simulink model "casperdemo"  (Simulink 6.2)
settings: Solver=ode45  StartTime=0.0  StopTime=16384  RelTol=1e-3
libraries: xbsIndex_r3 x1645, casper_library x163, testbench_lib x15, xps_library x1
(part 7 of 12)

== system casperdemo/Real FFT and Real PFB/fft_biplex_real_4x/biplex_core/fft_stage_3 ==
  in1 : Inport  Port=1  LatchInput=off
  in2 : Inport  Port=2  LatchInput=off
  of_in : Inport  Port=3  LatchInput=off
  sync : Inport  Port=4  LatchInput=off
  shift : Inport  Port=5  LatchInput=off
  Counter : xbsIndex_r3/Counter  cnt_type=Free Running  n_bits=FFTSize-FFTStage+1  bin_pt=0  arith_type=Unsigned  start_count=0  cnt_to=Inf  cnt_by_val=1  operation=Up  explicit_period=off  period=1  load_pin=off  rst=on  en=off  dbl_ovrd=off  show_param=off  use_rpm=off  gen_core=on
      settings: xl_area=[0, 0, 0, 0, 0, 0, 0]
  Delay : xbsIndex_r3/Delay  latency=1  reg_retiming=off  explicit_period=off  period=1  en=off  accept_only_valid=off  init_zero=on  dbl_ovrd=off  show_param=off
      settings: xl_area=[0, 0, 0, 0, 0, 0, 0]
  Logical1 : xbsIndex_r3/Logical  logical_function=OR  inputs=2  precision=Full  arith_type=Unsigned  n_bits=8  bin_pt=2  align_bp=on  latency=1  explicit_period=on  period=1  en=off  dbl_ovrd=off  show_param=off
      settings: xl_area=[0, 0, 0, 0, 0, 0, 0]
  Mux : xbsIndex_r3/Mux  inputs=2  precision=Full  arith_type="Signed  (2's comp)"  n_bits=8  bin_pt=2  quantization=Truncate  overflow=Wrap  latency=1  explicit_period=off  period=1  en=off  dbl_ovrd=off  show_param=off  mux_type=off  use_rpm=off  gen_core=on
      settings: xl_area=[0, 0, 0, 0, 0, 0, 0]
  Mux1 : xbsIndex_r3/Mux  inputs=2  precision=Full  arith_type="Signed  (2's comp)"  n_bits=8  bin_pt=2  quantization=Truncate  overflow=Wrap  latency=1  explicit_period=off  period=1  en=off  dbl_ovrd=off  show_param=off  mux_type=off  use_rpm=off  gen_core=on
      settings: xl_area=[0, 0, 0, 0, 0, 0, 0]
  Slice : xbsIndex_r3/Slice  Orientation=up  mode=Lower Bit Location + Width  nbits=1  bit1=-(FFTStage - 1)  base1=MSB of Input  bit0=FFTStage - 1  base0=LSB of Input  boolean_output=on  explicit_period=off  period=1  dbl_ovrd=off
  Slice1 : xbsIndex_r3/Slice  mode=Upper Bit Location + Width  nbits=1  bit1=0  base1=MSB of Input  bit0=0  base0=LSB of Input  boolean_output=off  explicit_period=off  period=1  dbl_ovrd=off
  butterfly_direct : Subsystem  AncestorBlock=casper_library/FFTs/butterfly_direct  mask(butterfly_direct){FFTSize=4, Coeffs=[0 1 2 3], StepPeriod=1, BitWidth=18, add_latency=2, mult_latency=3, bram_latency=2, use_bram=0, quantization=Truncate, overflow=Wrap}
      mask prompts: FFTSize "Size of FFT: (2^?)"; Coeffs "Coefficients: (0 to 2^(FFTSize-1)-1)"; StepPeriod "Coefficient Step Period: (2^?)"; BitWidth "Output Bitwidth:"; add_latency "Add Latency"; mult_latency "Mult Latency"; bram_latency "BRAM Latency"; use_bram "Store Coefficients in BRAM"; quantization "Quantization Behavior"; overflow "Overflow Behavior"
      mask init: same as casperdemo/Complex FFT and PFB with multiple simultaneous inputs/fft/fft_direct/butterfly1_0
      settings: AttributesFormatString=|
      | FFTSize=4, Coeffs=[0  1  2  3],
      |  StepPeriod=1, BitWidth=18
      mask StyleString: edit,edit,edit,edit,edit,edit,edit,edit,popup(Truncate|Round  (unbiased: +/- Inf)|Round  (unbiased: Even Values)),popup(Wrap|Saturate|Error)
  delay_b : Subsystem  BlockChoice=delay_slr
      link override delay_bram: bram_latency=bram_latency  DelayLen=2^(FFTSize-FFTStage)
      link override delay_slr: DelayLen=2^(FFTSize-FFTStage)
      settings: AttributesFormatString=%<BlockChoice>  TemplateBlock=casper_library/Delays/delay  MemberBlocks=delay_bram,delay_slr
  delay_f : Subsystem  BlockChoice=delay_slr
      link override delay_bram: bram_latency=bram_latency  DelayLen=2^(FFTSize-FFTStage)
      link override delay_slr: DelayLen=2^(FFTSize-FFTStage)
      settings: AttributesFormatString=%<BlockChoice>  TemplateBlock=casper_library/Delays/delay  MemberBlocks=delay_bram,delay_slr
  sync_delay : casper_library/Delays/sync_delay  DelayLen=2^(FFTSize - FFTStage)
      link override Constant: equ=P=C
      link override Constant1: equ=P=C
      link override Constant2: equ=P=C
      link override Constant3: equ=P=C
  out1 : Outport
  out2 : Outport  Port=2
  of : Outport  Port=3
  sync_out : Outport  Port=4
  wires:
  butterfly_direct/4(sync_out) -> sync_out/1
  butterfly_direct/1(a+bw) -> out1/1
  butterfly_direct/2(a-bw) -> out2/1
  butterfly_direct/3(of) -> Logical1/1
  Slice/1 -> butterfly_direct/4(shift)
  sync_delay/1 -> butterfly_direct/3(sync)
  delay_b/1(Out1) -> butterfly_direct/1(a)
  in2/1 -> delay_f/1(In1)
  Slice1/1 -> Mux1/1, Mux/1
  in1/1 -> Mux1/2, Mux/3
  delay_f/1(Out1) -> Mux/2, Mux1/3
  Mux1/1 -> delay_b/1(In1)
  Mux/1 -> butterfly_direct/2(b)
  Counter/1 -> Slice1/1
  sync/1 -> Delay/1, Counter/1
  Delay/1 -> sync_delay/1
  Logical1/1 -> of/1
  of_in/1 -> Logical1/2
  shift/1 -> Slice/1

== system casperdemo/Real FFT and Real PFB/fft_biplex_real_4x/biplex_core/fft_stage_4 ==
  in1 : Inport  Port=1  LatchInput=off
  in2 : Inport  Port=2  LatchInput=off
  of_in : Inport  Port=3  LatchInput=off
  sync : Inport  Port=4  LatchInput=off
  shift : Inport  Port=5  LatchInput=off
  Counter : xbsIndex_r3/Counter  cnt_type=Free Running  n_bits=FFTSize-FFTStage+1  bin_pt=0  arith_type=Unsigned  start_count=0  cnt_to=Inf  cnt_by_val=1  operation=Up  explicit_period=off  period=1  load_pin=off  rst=on  en=off  dbl_ovrd=off  show_param=off  use_rpm=off  gen_core=on
      settings: xl_area=[0, 0, 0, 0, 0, 0, 0]
  Delay : xbsIndex_r3/Delay  latency=1  reg_retiming=off  explicit_period=off  period=1  en=off  accept_only_valid=off  init_zero=on  dbl_ovrd=off  show_param=off
      settings: xl_area=[0, 0, 0, 0, 0, 0, 0]
  Logical1 : xbsIndex_r3/Logical  logical_function=OR  inputs=2  precision=Full  arith_type=Unsigned  n_bits=8  bin_pt=2  align_bp=on  latency=1  explicit_period=on  period=1  en=off  dbl_ovrd=off  show_param=off
      settings: xl_area=[0, 0, 0, 0, 0, 0, 0]
  Mux : xbsIndex_r3/Mux  inputs=2  precision=Full  arith_type="Signed  (2's comp)"  n_bits=8  bin_pt=2  quantization=Truncate  overflow=Wrap  latency=1  explicit_period=off  period=1  en=off  dbl_ovrd=off  show_param=off  mux_type=off  use_rpm=off  gen_core=on
      settings: xl_area=[0, 0, 0, 0, 0, 0, 0]
  Mux1 : xbsIndex_r3/Mux  inputs=2  precision=Full  arith_type="Signed  (2's comp)"  n_bits=8  bin_pt=2  quantization=Truncate  overflow=Wrap  latency=1  explicit_period=off  period=1  en=off  dbl_ovrd=off  show_param=off  mux_type=off  use_rpm=off  gen_core=on
      settings: xl_area=[0, 0, 0, 0, 0, 0, 0]
  Slice : xbsIndex_r3/Slice  Orientation=up  mode=Lower Bit Location + Width  nbits=1  bit1=-(FFTStage - 1)  base1=MSB of Input  bit0=FFTStage - 1  base0=LSB of Input  boolean_output=on  explicit_period=off  period=1  dbl_ovrd=off
  Slice1 : xbsIndex_r3/Slice  mode=Upper Bit Location + Width  nbits=1  bit1=0  base1=MSB of Input  bit0=0  base0=LSB of Input  boolean_output=off  explicit_period=off  period=1  dbl_ovrd=off
  butterfly_direct : Subsystem  AncestorBlock=casper_library/FFTs/butterfly_direct  mask(butterfly_direct){FFTSize=4, Coeffs=[0 1 2 3 4 5 6 7], StepPeriod=0, BitWidth=18, add_latency=2, mult_latency=3, bram_latency=2, use_bram=0, quantization=Truncate, overflow=Wrap}
      mask prompts: FFTSize "Size of FFT: (2^?)"; Coeffs "Coefficients: (0 to 2^(FFTSize-1)-1)"; StepPeriod "Coefficient Step Period: (2^?)"; BitWidth "Output Bitwidth:"; add_latency "Add Latency"; mult_latency "Mult Latency"; bram_latency "BRAM Latency"; use_bram "Store Coefficients in BRAM"; quantization "Quantization Behavior"; overflow "Overflow Behavior"
      mask init: same as casperdemo/Complex FFT and PFB with multiple simultaneous inputs/fft/fft_direct/butterfly1_0
      settings: AttributesFormatString=|
      | FFTSize=4, Coeffs=[0  1  2  3  4  5  6  7],
      |  StepPeriod=0, BitWidth=18
      mask StyleString: edit,edit,edit,edit,edit,edit,edit,edit,popup(Truncate|Round  (unbiased: +/- Inf)|Round  (unbiased: Even Values)),popup(Wrap|Saturate|Error)
  delay_b : Subsystem  BlockChoice=delay_slr
      link override delay_bram: bram_latency=bram_latency  DelayLen=2^(FFTSize-FFTStage)
      link override delay_slr: DelayLen=2^(FFTSize-FFTStage)
      settings: AttributesFormatString=%<BlockChoice>  TemplateBlock=casper_library/Delays/delay  MemberBlocks=delay_bram,delay_slr
  delay_f : Subsystem  BlockChoice=delay_slr
      link override delay_bram: bram_latency=bram_latency  DelayLen=2^(FFTSize-FFTStage)
      link override delay_slr: DelayLen=2^(FFTSize-FFTStage)
      settings: AttributesFormatString=%<BlockChoice>  TemplateBlock=casper_library/Delays/delay  MemberBlocks=delay_bram,delay_slr
  sync_delay : casper_library/Delays/sync_delay  DelayLen=2^(FFTSize - FFTStage)
      link override Constant: equ=P=C
      link override Constant1: equ=P=C
      link override Constant2: equ=P=C
      link override Constant3: equ=P=C
  out1 : Outport
  out2 : Outport  Port=2
  of : Outport  Port=3
  sync_out : Outport  Port=4
  wires:
  butterfly_direct/4(sync_out) -> sync_out/1
  butterfly_direct/1(a+bw) -> out1/1
  butterfly_direct/2(a-bw) -> out2/1
  butterfly_direct/3(of) -> Logical1/1
  Slice/1 -> butterfly_direct/4(shift)
  sync_delay/1 -> butterfly_direct/3(sync)
  delay_b/1(Out1) -> butterfly_direct/1(a)
  in2/1 -> delay_f/1(In1)
  Slice1/1 -> Mux1/1, Mux/1
  in1/1 -> Mux1/2, Mux/3
  delay_f/1(Out1) -> Mux/2, Mux1/3
  Mux1/1 -> delay_b/1(In1)
  Mux/1 -> butterfly_direct/2(b)
  Counter/1 -> Slice1/1
  sync/1 -> Delay/1, Counter/1
  Delay/1 -> sync_delay/1
  Logical1/1 -> of/1
  of_in/1 -> Logical1/2
  shift/1 -> Slice/1

== system casperdemo/Real FFT and Real PFB/pfb_fir_real/pol1_in1_first_tap/delay ==
  In1 : Inport  Port=1  LatchInput=off
  delay_bram : casper_library/Delays/delay_bram  DelayLen=2^(PFBSize-n_inputs)  bram_latency=bram_latency
  Out1 : Outport
  wires:
  In1/1 -> delay_bram/1
  delay_bram/1 -> Out1/1

== system casperdemo/Real FFT and Real PFB/pfb_fir_real/pol1_in1_first_tap/pfb_coeff_gen ==
  din : Inport  Port=1  LatchInput=off
  sync : Inport  Port=2  LatchInput=off
  Concat : xbsIndex_r3/Concat  num_inputs=4  explicit_period=off  period=1  dbl_ovrd=off
  Counter : xbsIndex_r3/Counter  cnt_type=Free Running  n_bits=4  bin_pt=0  arith_type=Unsigned  start_count=0  cnt_to=Inf  cnt_by_val=1  operation=Up  explicit_period=on  period=1  load_pin=off  rst=on  en=off  dbl_ovrd=off  show_param=off  use_rpm=on  gen_core=off
      settings: xl_area=[0, 0, 0, 0, 0, 0, 0]
  Delay : xbsIndex_r3/Delay  latency=bram_latency+1  reg_retiming=off  explicit_period=off  period=1  en=off  accept_only_valid=off  init_zero=on  dbl_ovrd=off  show_param=off
      settings: xl_area=[0, 0, 0, 0, 0, 0, 0]
  Delay1 : xbsIndex_r3/Delay  latency=3  reg_retiming=off  explicit_period=off  period=1  en=off  accept_only_valid=off  init_zero=on  dbl_ovrd=off  show_param=off
      settings: xl_area=[0, 0, 0, 0, 0, 0, 0]
  ROM1 : xbsIndex_r3/ROM  depth=16  initVector=[-3.1185374660155e-018 -0.00263735909580334 -0.00578984434733957 -0.0097994723321974 -0.0149350827451364 -0.021332873381912 -0.0289429297169117 -0.0374871259095755 -0.0464331498505763 -0.054988365242619 -0.0621158358774173 -0.0665731978343029 -0.0669732935066947 -0.0618637102387744 -0.0498207328553067 -0.0295518537627434]  arith_type="Signed  (2's comp)"  n_bits=8  bin_pt=7  latency=2  init_zero=on  explicit_period=off  period=1  rst=off  init_reg=0  en=off  dbl_ovrd=off  show_param=on  distributed_mem=on  use_rpm=on  gen_core=off
      settings: xl_area=[0, 0, 0, 0, 0, 0, 0]
  ROM2 : xbsIndex_r3/ROM  depth=16  initVector=[2.14971748489781e-017 0.039557878919974 0.0894252110701411 0.149419992109658 0.218834505309546 0.29642479737618 0.380432267164858 0.468637627642037 0.558445322336343 0.646994370487006 0.731289732081715 0.808346763068111 0.875340286111191 0.929749314368444 0.969488576724053 0.993018702047571]  arith_type="Signed  (2's comp)"  n_bits=8  bin_pt=7  latency=2  init_zero=on  explicit_period=off  period=1  rst=off  init_reg=0  en=off  dbl_ovrd=off  show_param=on  distributed_mem=on  use_rpm=on  gen_core=off
      settings: xl_area=[0, 0, 0, 0, 0, 0, 0]
  ROM3 : xbsIndex_r3/ROM  depth=16  initVector=[0.999428183760704 0.988481980811812 0.960633699526478 0.917000599560915 0.859303017901024 0.789772045316812 0.711031265694996 0.625959945208598 0.537546129240986 0.448738600765768 0.36230654625236 0.280715079012005 0.20602354182225 0.139811844485469 0.0831381115043222 0.0365287647378851]  arith_type="Signed  (2's comp)"  n_bits=8  bin_pt=7  latency=2  init_zero=on  explicit_period=off  period=1  rst=off  init_reg=0  en=off  dbl_ovrd=off  show_param=off  distributed_mem=on  use_rpm=on  gen_core=off
      settings: xl_area=[0, 0, 0, 0, 0, 0, 0]
  ROM4 : xbsIndex_r3/ROM  depth=16  initVector=[1.9710098464648e-017 -0.0268924122607391 -0.0449798239071789 -0.0553900832155681 -0.0594466434903448 -0.0585648122922967 -0.0541523577793221 -0.0475209911960375 -0.0398141063792136 -0.0319546763151778 -0.0246155042127458 -0.0182122364356803 -0.0129178040136007 -0.00869539776353592 -0.00534581149262307 -0.00256409509972699]  arith_type="Signed  (2's comp)"  n_bits=8  bin_pt=7  latency=2  init_zero=on  explicit_period=off  period=1  rst=off  init_reg=0  en=off  dbl_ovrd=off  show_param=off  distributed_mem=on  use_rpm=on  gen_core=off
      settings: xl_area=[0, 0, 0, 0, 0, 0, 0]
  Register : xbsIndex_r3/Register  init=0  reg_only_valid=off  explicit_period=off  period=1  rst=off  en=off  out_en=off  dbl_ovrd=off  show_param=off
      settings: xl_area=[0, 0, 0, 0, 0, 0, 0]
  Reinterpret{1..4} (4 alike) : xbsIndex_r3/Reinterpret  force_arith_type=on  arith_type=Unsigned  force_bin_pt=on  bin_pt=0  force_valid=on
  dout : Outport
  sync_out : Outport  Port=2
  coeff : Outport  Port=3
  wires:
  din/1 -> Delay1/1
  Delay1/1 -> dout/1
  sync/1 -> Counter/1, Delay/1
  Delay/1 -> sync_out/1
  Concat/1 -> Register/1
  Register/1 -> coeff/1
  Counter/1 -> ROM1/1, ROM2/1, ROM3/1, ROM4/1
  ROM1/1 -> Reinterpret1/1
  Reinterpret1/1 -> Concat/1
  ROM2/1 -> Reinterpret2/1
  Reinterpret2/1 -> Concat/2
  ROM3/1 -> Reinterpret3/1
  Reinterpret3/1 -> Concat/3
  ROM4/1 -> Reinterpret4/1
  Reinterpret4/1 -> Concat/4

== system casperdemo/Real FFT and Real PFB/pfb_fir_real/pol1_in1_last_tap/pfb_real_add_tree ==
  din : Inport  Port=1  LatchInput=off
  sync : Inport  Port=2  LatchInput=off
  Reint{0..3} (4 alike) : xbsIndex_r3/Reinterpret  force_arith_type=on  arith_type="Signed  (2's comp)"  force_bin_pt=on  bin_pt=CoeffBitWidth + BitWidthIn - 2  force_valid=on
  Slice0 : xbsIndex_r3/Slice  mode=Upper Bit Location + Width  nbits=CoeffBitWidth + BitWidthIn  bit1=-0*(CoeffBitWidth + BitWidthIn)  base1=MSB of Input  bit0=0  base0=MSB of Input  boolean_output=off  explicit_period=off  period=1  dbl_ovrd=off
  Slice1 : xbsIndex_r3/Slice  mode=Upper Bit Location + Width  nbits=CoeffBitWidth + BitWidthIn  bit1=-1*(CoeffBitWidth + BitWidthIn)  base1=MSB of Input  bit0=0  base0=MSB of Input  boolean_output=off  explicit_period=off  period=1  dbl_ovrd=off
  Slice2 : xbsIndex_r3/Slice  mode=Upper Bit Location + Width  nbits=CoeffBitWidth + BitWidthIn  bit1=-2*(CoeffBitWidth + BitWidthIn)  base1=MSB of Input  bit0=0  base0=MSB of Input  boolean_output=off  explicit_period=off  period=1  dbl_ovrd=off
  Slice3 : xbsIndex_r3/Slice  mode=Upper Bit Location + Width  nbits=CoeffBitWidth + BitWidthIn  bit1=-3*(CoeffBitWidth + BitWidthIn)  base1=MSB of Input  bit0=0  base0=MSB of Input  boolean_output=off  explicit_period=off  period=1  dbl_ovrd=off
  adder_tree1 : Subsystem  AncestorBlock=casper_library/Misc/adder_tree  mask(adder_tree){n_inputs=4, latency=1}
      mask prompts: n_inputs "Number of Inputs"; latency "Add Latency"
      mask help: Sums all inputs using a tree of adds and delays.
      mask init:
      | adder_tree_init(gcb, ...
      |     'n_inputs', n_inputs, ...
      |     'latency', latency);
      settings: AttributesFormatString=latency 2
      mask Help: eval('xlWeb([getenv(''MLIB_ROOT''), ''\doc\html\sp_adder_tree\sp_adder_tree.html''])')
  convert1 : xbsIndex_r3/Convert  arith_type="Signed  (2's comp)"  n_bits=BitWidthOut  bin_pt=BitWidthOut-1  quantization=Truncate  overflow=Saturate  latency=add_latency  explicit_period=off  period=1  dbl_ovrd=off  show_param=off  inserted_by_tool=off  pipeline=off
      settings: xl_area=[0, 0, 0, 0, 0, 0, 0]
  delay1 : xbsIndex_r3/Delay  latency=1  reg_retiming=off  explicit_period=off  period=1  en=off  accept_only_valid=off  init_zero=on  dbl_ovrd=off  show_param=off
      settings: xl_area=[0, 0, 0, 0, 0, 0, 0]
  scale1 : xbsIndex_r3/Scale  scale_factor=-3  explicit_period=off  period=1  dbl_ovrd=off
  dout : Outport
  sync_out : Outport  Port=2
  wires:
  adder_tree1/2(dout) -> scale1/1
  scale1/1 -> convert1/1
  convert1/1 -> dout/1
  sync/1 -> adder_tree1/1(sync)
  adder_tree1/1(sync_out) -> delay1/1
  delay1/1 -> sync_out/1
  din/1 -> Slice0/1, Slice1/1, Slice2/1, Slice3/1
  Slice0/1 -> Reint0/1
  Reint0/1 -> adder_tree1/2(din1)
  Slice1/1 -> Reint1/1
  Reint1/1 -> adder_tree1/3(din2)
  Slice2/1 -> Reint2/1
  Reint2/1 -> adder_tree1/4(din3)
  Slice3/1 -> Reint3/1
  Reint3/1 -> adder_tree1/5(din4)

== system casperdemo/Complex FFT and PFB/fft/fft_biplex0/biplex_core/fft_stage_1 ==
  in1 : Inport  Port=1  LatchInput=off
  in2 : Inport  Port=2  LatchInput=off
  sync : Inport  Port=3  LatchInput=off
  shift : Inport  Port=4  LatchInput=off
  Counter : xbsIndex_r3/Counter  cnt_type=Free Running  n_bits=FFTSize-FFTStage+1  bin_pt=0  arith_type=Unsigned  start_count=0  cnt_to=Inf  cnt_by_val=1  operation=Up  explicit_period=off  period=1  load_pin=off  rst=on  en=off  dbl_ovrd=off  show_param=off  use_rpm=off  gen_core=on
      settings: xl_area=[0, 0, 0, 0, 0, 0, 0]
  Delay : xbsIndex_r3/Delay  latency=1  reg_retiming=off  explicit_period=off  period=1  en=off  accept_only_valid=off  init_zero=on  dbl_ovrd=off  show_param=off
      settings: xl_area=[0, 0, 0, 0, 0, 0, 0]
  Mux : xbsIndex_r3/Mux  inputs=2  precision=Full  arith_type="Signed  (2's comp)"  n_bits=8  bin_pt=2  quantization=Truncate  overflow=Wrap  latency=1  explicit_period=off  period=1  en=off  dbl_ovrd=off  show_param=off  mux_type=off  use_rpm=off  gen_core=on
      settings: xl_area=[0, 0, 0, 0, 0, 0, 0]
  Mux1 : xbsIndex_r3/Mux  inputs=2  precision=Full  arith_type="Signed  (2's comp)"  n_bits=8  bin_pt=2  quantization=Truncate  overflow=Wrap  latency=1  explicit_period=off  period=1  en=off  dbl_ovrd=off  show_param=off  mux_type=off  use_rpm=off  gen_core=on
      settings: xl_area=[0, 0, 0, 0, 0, 0, 0]
  Slice : xbsIndex_r3/Slice  Orientation=up  mode=Lower Bit Location + Width  nbits=1  bit1=-(FFTStage - 1)  base1=MSB of Input  bit0=FFTStage - 1  base0=LSB of Input  boolean_output=on  explicit_period=off  period=1  dbl_ovrd=off
  Slice1 : xbsIndex_r3/Slice  mode=Upper Bit Location + Width  nbits=1  bit1=0  base1=MSB of Input  bit0=0  base0=LSB of Input  boolean_output=off  explicit_period=off  period=1  dbl_ovrd=off
  butterfly : Subsystem
  delay_b : Subsystem  BlockChoice=delay_slr
      link override delay_bram: bram_latency=bram_latency  DelayLen=2^(FFTSize-FFTStage)
      link override delay_bram/Constant2: equ=P=C
      link override delay_slr: DelayLen=2^(FFTSize-FFTStage)
      settings: AttributesFormatString=%<BlockChoice>  TemplateBlock=casper_library/Delays/delay  MemberBlocks=delay_bram,delay_slr
  delay_f : Subsystem  BlockChoice=delay_slr
      link override delay_bram: bram_latency=bram_latency  DelayLen=2^(FFTSize-FFTStage)
      link override delay_bram/Constant2: equ=P=C
      link override delay_slr: DelayLen=2^(FFTSize-FFTStage)
      settings: AttributesFormatString=%<BlockChoice>  TemplateBlock=casper_library/Delays/delay  MemberBlocks=delay_bram,delay_slr
  sync_delay : casper_library/Delays/sync_delay  DelayLen=2^(FFTSize - FFTStage)
      link override Constant: equ=P=C
      link override Constant1: equ=P=C
      link override Constant2: equ=P=C
      link override Constant3: equ=P=C
  out1 : Outport
  out2 : Outport  Port=2
  of : Outport  Port=3
  sync_out : Outport  Port=4
  wires:
  shift/1 -> Slice/1
  Delay/1 -> sync_delay/1
  sync/1 -> Counter/1, Delay/1
  Counter/1 -> Slice1/1
  Mux/1 -> butterfly/2(b)
  Mux1/1 -> delay_b/1(In1)
  delay_f/1(Out1) -> Mux1/3, Mux/2
  in1/1 -> Mux/3, Mux1/2
  Slice1/1 -> Mux/1, Mux1/1
  in2/1 -> delay_f/1(In1)
  delay_b/1(Out1) -> butterfly/1(a)
  sync_delay/1 -> butterfly/3(sync)
  Slice/1 -> butterfly/4(shift)
  butterfly/3(of) -> of/1
  butterfly/2(a-bw) -> out2/1
  butterfly/1(a+bw) -> out1/1
  butterfly/4(sync_out) -> sync_out/1

== system casperdemo/Complex FFT and PFB/fft/fft_biplex0/biplex_core/fft_stage_2 ==
  in1 : Inport  Port=1  LatchInput=off
  in2 : Inport  Port=2  LatchInput=off
  of_in : Inport  Port=3  LatchInput=off
  sync : Inport  Port=4  LatchInput=off
  shift : Inport  Port=5  LatchInput=off
  Counter : xbsIndex_r3/Counter  cnt_type=Free Running  n_bits=FFTSize-FFTStage+1  bin_pt=0  arith_type=Unsigned  start_count=0  cnt_to=Inf  cnt_by_val=1  operation=Up  explicit_period=off  period=1  load_pin=off  rst=on  en=off  dbl_ovrd=off  show_param=off  use_rpm=off  gen_core=on
      settings: xl_area=[0, 0, 0, 0, 0, 0, 0]
  Delay : xbsIndex_r3/Delay  latency=1  reg_retiming=off  explicit_period=off  period=1  en=off  accept_only_valid=off  init_zero=on  dbl_ovrd=off  show_param=off
      settings: xl_area=[0, 0, 0, 0, 0, 0, 0]
  Logical1 : xbsIndex_r3/Logical  logical_function=OR  inputs=2  precision=Full  arith_type=Unsigned  n_bits=8  bin_pt=2  align_bp=on  latency=1  explicit_period=on  period=1  en=off  dbl_ovrd=off  show_param=off
      settings: xl_area=[0, 0, 0, 0, 0, 0, 0]
  Mux : xbsIndex_r3/Mux  inputs=2  precision=Full  arith_type="Signed  (2's comp)"  n_bits=8  bin_pt=2  quantization=Truncate  overflow=Wrap  latency=1  explicit_period=off  period=1  en=off  dbl_ovrd=off  show_param=off  mux_type=off  use_rpm=off  gen_core=on
      settings: xl_area=[0, 0, 0, 0, 0, 0, 0]
  Mux1 : xbsIndex_r3/Mux  inputs=2  precision=Full  arith_type="Signed  (2's comp)"  n_bits=8  bin_pt=2  quantization=Truncate  overflow=Wrap  latency=1  explicit_period=off  period=1  en=off  dbl_ovrd=off  show_param=off  mux_type=off  use_rpm=off  gen_core=on
      settings: xl_area=[0, 0, 0, 0, 0, 0, 0]
  Slice : xbsIndex_r3/Slice  Orientation=up  mode=Lower Bit Location + Width  nbits=1  bit1=-(FFTStage - 1)  base1=MSB of Input  bit0=FFTStage - 1  base0=LSB of Input  boolean_output=on  explicit_period=off  period=1  dbl_ovrd=off
  Slice1 : xbsIndex_r3/Slice  mode=Upper Bit Location + Width  nbits=1  bit1=0  base1=MSB of Input  bit0=0  base0=LSB of Input  boolean_output=off  explicit_period=off  period=1  dbl_ovrd=off
  butterfly_direct : Subsystem  AncestorBlock=casper_library/FFTs/butterfly_direct  mask(butterfly_direct){FFTSize=4, Coeffs=[0 1], StepPeriod=2, BitWidth=18, add_latency=2, mult_latency=3, bram_latency=2, use_bram=0, quantization=Truncate, overflow=Wrap}
      mask prompts: FFTSize "Size of FFT: (2^?)"; Coeffs "Coefficients: (0 to 2^(FFTSize-1)-1)"; StepPeriod "Coefficient Step Period: (2^?)"; BitWidth "Output Bitwidth:"; add_latency "Add Latency"; mult_latency "Mult Latency"; bram_latency "BRAM Latency"; use_bram "Store Coefficients in BRAM"; quantization "Quantization Behavior"; overflow "Overflow Behavior"
      mask init: same as casperdemo/Complex FFT and PFB with multiple simultaneous inputs/fft/fft_direct/butterfly1_0
      settings: AttributesFormatString=|
      | FFTSize=4, Coeffs=[0  1],
      |  StepPeriod=2, BitWidth=18
      mask StyleString: edit,edit,edit,edit,edit,edit,edit,edit,popup(Truncate|Round  (unbiased: +/- Inf)|Round  (unbiased: Even Values)),popup(Wrap|Saturate|Error)
  delay_b : Subsystem  BlockChoice=delay_slr
      link override delay_bram: bram_latency=bram_latency  DelayLen=2^(FFTSize-FFTStage)
      link override delay_bram/Constant2: equ=P=C
      link override delay_slr: DelayLen=2^(FFTSize-FFTStage)
      settings: AttributesFormatString=%<BlockChoice>  TemplateBlock=casper_library/Delays/delay  MemberBlocks=delay_bram,delay_slr
  delay_f : Subsystem  BlockChoice=delay_slr
      link override delay_bram: bram_latency=bram_latency  DelayLen=2^(FFTSize-FFTStage)
      link override delay_bram/Constant2: equ=P=C
      link override delay_slr: DelayLen=2^(FFTSize-FFTStage)
      settings: AttributesFormatString=%<BlockChoice>  TemplateBlock=casper_library/Delays/delay  MemberBlocks=delay_bram,delay_slr
  sync_delay : casper_library/Delays/sync_delay  DelayLen=2^(FFTSize - FFTStage)
      link override Constant: equ=P=C
      link override Constant1: equ=P=C
      link override Constant2: equ=P=C
      link override Constant3: equ=P=C
  out1 : Outport
  out2 : Outport  Port=2
  of : Outport  Port=3
  sync_out : Outport  Port=4
  wires:
  butterfly_direct/4(sync_out) -> sync_out/1
  butterfly_direct/1(a+bw) -> out1/1
  butterfly_direct/2(a-bw) -> out2/1
  butterfly_direct/3(of) -> Logical1/1
  Slice/1 -> butterfly_direct/4(shift)
  sync_delay/1 -> butterfly_direct/3(sync)
  delay_b/1(Out1) -> butterfly_direct/1(a)
  in2/1 -> delay_f/1(In1)
  Slice1/1 -> Mux1/1, Mux/1
  in1/1 -> Mux1/2, Mux/3
  delay_f/1(Out1) -> Mux/2, Mux1/3
  Mux1/1 -> delay_b/1(In1)
  Mux/1 -> butterfly_direct/2(b)
  Counter/1 -> Slice1/1
  sync/1 -> Delay/1, Counter/1
  Delay/1 -> sync_delay/1
  Logical1/1 -> of/1
  of_in/1 -> Logical1/2
  shift/1 -> Slice/1

== system casperdemo/Complex FFT and PFB/fft/fft_biplex0/biplex_core/fft_stage_3 ==
  in1 : Inport  Port=1  LatchInput=off
  in2 : Inport  Port=2  LatchInput=off
  of_in : Inport  Port=3  LatchInput=off
  sync : Inport  Port=4  LatchInput=off
  shift : Inport  Port=5  LatchInput=off
  Counter : xbsIndex_r3/Counter  cnt_type=Free Running  n_bits=FFTSize-FFTStage+1  bin_pt=0  arith_type=Unsigned  start_count=0  cnt_to=Inf  cnt_by_val=1  operation=Up  explicit_period=off  period=1  load_pin=off  rst=on  en=off  dbl_ovrd=off  show_param=off  use_rpm=off  gen_core=on
      settings: xl_area=[0, 0, 0, 0, 0, 0, 0]
  Delay : xbsIndex_r3/Delay  latency=1  reg_retiming=off  explicit_period=off  period=1  en=off  accept_only_valid=off  init_zero=on  dbl_ovrd=off  show_param=off
      settings: xl_area=[0, 0, 0, 0, 0, 0, 0]
  Logical1 : xbsIndex_r3/Logical  logical_function=OR  inputs=2  precision=Full  arith_type=Unsigned  n_bits=8  bin_pt=2  align_bp=on  latency=1  explicit_period=on  period=1  en=off  dbl_ovrd=off  show_param=off
      settings: xl_area=[0, 0, 0, 0, 0, 0, 0]
  Mux : xbsIndex_r3/Mux  inputs=2  precision=Full  arith_type="Signed  (2's comp)"  n_bits=8  bin_pt=2  quantization=Truncate  overflow=Wrap  latency=1  explicit_period=off  period=1  en=off  dbl_ovrd=off  show_param=off  mux_type=off  use_rpm=off  gen_core=on
      settings: xl_area=[0, 0, 0, 0, 0, 0, 0]
  Mux1 : xbsIndex_r3/Mux  inputs=2  precision=Full  arith_type="Signed  (2's comp)"  n_bits=8  bin_pt=2  quantization=Truncate  overflow=Wrap  latency=1  explicit_period=off  period=1  en=off  dbl_ovrd=off  show_param=off  mux_type=off  use_rpm=off  gen_core=on
      settings: xl_area=[0, 0, 0, 0, 0, 0, 0]
  Slice : xbsIndex_r3/Slice  Orientation=up  mode=Lower Bit Location + Width  nbits=1  bit1=-(FFTStage - 1)  base1=MSB of Input  bit0=FFTStage - 1  base0=LSB of Input  boolean_output=on  explicit_period=off  period=1  dbl_ovrd=off
  Slice1 : xbsIndex_r3/Slice  mode=Upper Bit Location + Width  nbits=1  bit1=0  base1=MSB of Input  bit0=0  base0=LSB of Input  boolean_output=off  explicit_period=off  period=1  dbl_ovrd=off
  butterfly_direct : Subsystem  AncestorBlock=casper_library/FFTs/butterfly_direct  mask(butterfly_direct){FFTSize=4, Coeffs=[0 1 2 3], StepPeriod=1, BitWidth=18, add_latency=2, mult_latency=3, bram_latency=2, use_bram=0, quantization=Truncate, overflow=Wrap}
      mask prompts: FFTSize "Size of FFT: (2^?)"; Coeffs "Coefficients: (0 to 2^(FFTSize-1)-1)"; StepPeriod "Coefficient Step Period: (2^?)"; BitWidth "Output Bitwidth:"; add_latency "Add Latency"; mult_latency "Mult Latency"; bram_latency "BRAM Latency"; use_bram "Store Coefficients in BRAM"; quantization "Quantization Behavior"; overflow "Overflow Behavior"
      mask init: same as casperdemo/Complex FFT and PFB with multiple simultaneous inputs/fft/fft_direct/butterfly1_0
      settings: AttributesFormatString=|
      | FFTSize=4, Coeffs=[0  1  2  3],
      |  StepPeriod=1, BitWidth=18
      mask StyleString: edit,edit,edit,edit,edit,edit,edit,edit,popup(Truncate|Round  (unbiased: +/- Inf)|Round  (unbiased: Even Values)),popup(Wrap|Saturate|Error)
  delay_b : Subsystem  BlockChoice=delay_slr
      link override delay_bram: bram_latency=bram_latency  DelayLen=2^(FFTSize-FFTStage)
      link override delay_slr: DelayLen=2^(FFTSize-FFTStage)
      settings: AttributesFormatString=%<BlockChoice>  TemplateBlock=casper_library/Delays/delay  MemberBlocks=delay_bram,delay_slr
  delay_f : Subsystem  BlockChoice=delay_slr
      link override delay_bram: bram_latency=bram_latency  DelayLen=2^(FFTSize-FFTStage)
      link override delay_slr: DelayLen=2^(FFTSize-FFTStage)
      settings: AttributesFormatString=%<BlockChoice>  TemplateBlock=casper_library/Delays/delay  MemberBlocks=delay_bram,delay_slr
  sync_delay : casper_library/Delays/sync_delay  DelayLen=2^(FFTSize - FFTStage)
      link override Constant: equ=P=C
      link override Constant1: equ=P=C
      link override Constant2: equ=P=C
      link override Constant3: equ=P=C
  out1 : Outport
  out2 : Outport  Port=2
  of : Outport  Port=3
  sync_out : Outport  Port=4
  wires:
  butterfly_direct/4(sync_out) -> sync_out/1
  butterfly_direct/1(a+bw) -> out1/1
  butterfly_direct/2(a-bw) -> out2/1
  butterfly_direct/3(of) -> Logical1/1
  Slice/1 -> butterfly_direct/4(shift)
  sync_delay/1 -> butterfly_direct/3(sync)
  delay_b/1(Out1) -> butterfly_direct/1(a)
  in2/1 -> delay_f/1(In1)
  Slice1/1 -> Mux1/1, Mux/1
  in1/1 -> Mux1/2, Mux/3
  delay_f/1(Out1) -> Mux/2, Mux1/3
  Mux1/1 -> delay_b/1(In1)
  Mux/1 -> butterfly_direct/2(b)
  Counter/1 -> Slice1/1
  sync/1 -> Delay/1, Counter/1
  Delay/1 -> sync_delay/1
  Logical1/1 -> of/1
  of_in/1 -> Logical1/2
  shift/1 -> Slice/1

== system casperdemo/Complex FFT and PFB/fft/fft_biplex0/biplex_core/fft_stage_4 ==
  in1 : Inport  Port=1  LatchInput=off
  in2 : Inport  Port=2  LatchInput=off
  of_in : Inport  Port=3  LatchInput=off
  sync : Inport  Port=4  LatchInput=off
  shift : Inport  Port=5  LatchInput=off
  Counter : xbsIndex_r3/Counter  cnt_type=Free Running  n_bits=FFTSize-FFTStage+1  bin_pt=0  arith_type=Unsigned  start_count=0  cnt_to=Inf  cnt_by_val=1  operation=Up  explicit_period=off  period=1  load_pin=off  rst=on  en=off  dbl_ovrd=off  show_param=off  use_rpm=off  gen_core=on
      settings: xl_area=[0, 0, 0, 0, 0, 0, 0]
  Delay : xbsIndex_r3/Delay  latency=1  reg_retiming=off  explicit_period=off  period=1  en=off  accept_only_valid=off  init_zero=on  dbl_ovrd=off  show_param=off
      settings: xl_area=[0, 0, 0, 0, 0, 0, 0]
  Logical1 : xbsIndex_r3/Logical  logical_function=OR  inputs=2  precision=Full  arith_type=Unsigned  n_bits=8  bin_pt=2  align_bp=on  latency=1  explicit_period=on  period=1  en=off  dbl_ovrd=off  show_param=off
      settings: xl_area=[0, 0, 0, 0, 0, 0, 0]
  Mux : xbsIndex_r3/Mux  inputs=2  precision=Full  arith_type="Signed  (2's comp)"  n_bits=8  bin_pt=2  quantization=Truncate  overflow=Wrap  latency=1  explicit_period=off  period=1  en=off  dbl_ovrd=off  show_param=off  mux_type=off  use_rpm=off  gen_core=on
      settings: xl_area=[0, 0, 0, 0, 0, 0, 0]
  Mux1 : xbsIndex_r3/Mux  inputs=2  precision=Full  arith_type="Signed  (2's comp)"  n_bits=8  bin_pt=2  quantization=Truncate  overflow=Wrap  latency=1  explicit_period=off  period=1  en=off  dbl_ovrd=off  show_param=off  mux_type=off  use_rpm=off  gen_core=on
      settings: xl_area=[0, 0, 0, 0, 0, 0, 0]
  Slice : xbsIndex_r3/Slice  Orientation=up  mode=Lower Bit Location + Width  nbits=1  bit1=-(FFTStage - 1)  base1=MSB of Input  bit0=FFTStage - 1  base0=LSB of Input  boolean_output=on  explicit_period=off  period=1  dbl_ovrd=off
  Slice1 : xbsIndex_r3/Slice  mode=Upper Bit Location + Width  nbits=1  bit1=0  base1=MSB of Input  bit0=0  base0=LSB of Input  boolean_output=off  explicit_period=off  period=1  dbl_ovrd=off
  butterfly_direct : Subsystem  AncestorBlock=casper_library/FFTs/butterfly_direct  mask(butterfly_direct){FFTSize=4, Coeffs=[0 1 2 3 4 5 6 7], StepPeriod=0, BitWidth=18, add_latency=2, mult_latency=3, bram_latency=2, use_bram=0, quantization=Truncate, overflow=Wrap}
      mask prompts: FFTSize "Size of FFT: (2^?)"; Coeffs "Coefficients: (0 to 2^(FFTSize-1)-1)"; StepPeriod "Coefficient Step Period: (2^?)"; BitWidth "Output Bitwidth:"; add_latency "Add Latency"; mult_latency "Mult Latency"; bram_latency "BRAM Latency"; use_bram "Store Coefficients in BRAM"; quantization "Quantization Behavior"; overflow "Overflow Behavior"
      mask init: same as casperdemo/Complex FFT and PFB with multiple simultaneous inputs/fft/fft_direct/butterfly1_0
      settings: AttributesFormatString=|
      | FFTSize=4, Coeffs=[0  1  2  3  4  5  6  7],
      |  StepPeriod=0, BitWidth=18
      mask StyleString: edit,edit,edit,edit,edit,edit,edit,edit,popup(Truncate|Round  (unbiased: +/- Inf)|Round  (unbiased: Even Values)),popup(Wrap|Saturate|Error)
  delay_b : Subsystem  BlockChoice=delay_slr
      link override delay_bram: bram_latency=bram_latency  DelayLen=2^(FFTSize-FFTStage)
      link override delay_slr: DelayLen=2^(FFTSize-FFTStage)
      settings: AttributesFormatString=%<BlockChoice>  TemplateBlock=casper_library/Delays/delay  MemberBlocks=delay_bram,delay_slr
  delay_f : Subsystem  BlockChoice=delay_slr
      link override delay_bram: bram_latency=bram_latency  DelayLen=2^(FFTSize-FFTStage)
      link override delay_slr: DelayLen=2^(FFTSize-FFTStage)
      settings: AttributesFormatString=%<BlockChoice>  TemplateBlock=casper_library/Delays/delay  MemberBlocks=delay_bram,delay_slr
  sync_delay : casper_library/Delays/sync_delay  DelayLen=2^(FFTSize - FFTStage)
      link override Constant: equ=P=C
      link override Constant1: equ=P=C
      link override Constant2: equ=P=C
      link override Constant3: equ=P=C
  out1 : Outport
  out2 : Outport  Port=2
  of : Outport  Port=3
  sync_out : Outport  Port=4
  wires:
  butterfly_direct/4(sync_out) -> sync_out/1
  butterfly_direct/1(a+bw) -> out1/1
  butterfly_direct/2(a-bw) -> out2/1
  butterfly_direct/3(of) -> Logical1/1
  Slice/1 -> butterfly_direct/4(shift)
  sync_delay/1 -> butterfly_direct/3(sync)
  delay_b/1(Out1) -> butterfly_direct/1(a)
  in2/1 -> delay_f/1(In1)
  Slice1/1 -> Mux1/1, Mux/1
  in1/1 -> Mux1/2, Mux/3
  delay_f/1(Out1) -> Mux/2, Mux1/3
  Mux1/1 -> delay_b/1(In1)
  Mux/1 -> butterfly_direct/2(b)
  Counter/1 -> Slice1/1
  sync/1 -> Delay/1, Counter/1
  Delay/1 -> sync_delay/1
  Logical1/1 -> of/1
  of_in/1 -> Logical1/2
  shift/1 -> Slice/1

== system casperdemo/Complex FFT and PFB/fft/fft_biplex0/biplex_cplx_unscrambler/reorder ==
  sync : Inport  Port=1  LatchInput=off
  en : Inport  Port=2  LatchInput=off
  din0 : Inport  Port=3  LatchInput=off
  Counter : xbsIndex_r3/Counter  cnt_type=Count Limited  n_bits=5  bin_pt=0  arith_type=Unsigned  start_count=0  cnt_to=31  cnt_by_val=1  operation=Up  explicit_period=off  period=1  load_pin=off  rst=on  en=on  dbl_ovrd=off  show_param=off  use_rpm=on  gen_core=off
      settings: xl_area=[0, 0, 0, 0, 0, 0, 0]
  Mux : xbsIndex_r3/Mux  inputs=2  precision=Full  arith_type="Signed  (2's comp)"  n_bits=8  bin_pt=2  quantization=Truncate  overflow=Wrap  latency=1  explicit_period=off  period=1  en=off  dbl_ovrd=off  show_param=off  mux_type=off  use_rpm=off  gen_core=off
      settings: xl_area=[0, 0, 0, 0, 0, 0, 0]
  Slice1 : xbsIndex_r3/Slice  mode=Upper Bit Location + Width  nbits=1  bit1=0  base1=MSB of Input  bit0=0  base0=LSB of Input  boolean_output=off  explicit_period=off  period=1  dbl_ovrd=off
  Slice2 : xbsIndex_r3/Slice  mode=Lower Bit Location + Width  nbits=4  bit1=0  base1=MSB of Input  bit0=0  base0=LSB of Input  boolean_output=off  explicit_period=off  period=1  dbl_ovrd=off
  bram0 : xbsIndex_r3/Single Port RAM  depth=16  initVector=sin(pi*(0:15)/16)  write_mode=Read Before Write  latency=2  init_zero=on  explicit_period=off  period=1  rst=off  init_reg=0  en=off  dbl_ovrd=off  show_param=off  distributed_mem=off  use_rpm=off  gen_core=off
      settings: xl_area=[0, 0, 0, 0, 0, 0, 0]
  delay_d0 : xbsIndex_r3/Delay  latency=0  reg_retiming=off  explicit_period=off  period=1  en=off  accept_only_valid=off  init_zero=on  dbl_ovrd=off  show_param=off
      settings: xl_area=[0, 0, 0, 0, 0, 0, 0]
  delay_din0 : xbsIndex_r3/Delay  latency=1  reg_retiming=off  explicit_period=off  period=1  en=off  accept_only_valid=off  init_zero=on  dbl_ovrd=off  show_param=off
      settings: xl_area=[0, 0, 0, 0, 0, 0, 0]
  delay_map1 : xbsIndex_r3/Delay  latency=0*map_latency  reg_retiming=off  explicit_period=off  period=1  en=off  accept_only_valid=off  init_zero=on  dbl_ovrd=off  show_param=off
      settings: xl_area=[0, 0, 0, 0, 0, 0, 0]
  delay_sel : xbsIndex_r3/Delay  latency=0  reg_retiming=off  explicit_period=off  period=1  en=off  accept_only_valid=off  init_zero=on  dbl_ovrd=off  show_param=off
      settings: xl_area=[0, 0, 0, 0, 0, 0, 0]
  delay_valid : xbsIndex_r3/Delay  latency=3  reg_retiming=off  explicit_period=off  period=1  en=off  accept_only_valid=off  init_zero=on  dbl_ovrd=off  show_param=off
      settings: xl_area=[0, 0, 0, 0, 0, 0, 0]
  delay_we : xbsIndex_r3/Delay  latency=0  reg_retiming=off  explicit_period=off  period=1  en=off  accept_only_valid=off  init_zero=on  dbl_ovrd=off  show_param=off
      settings: xl_area=[0, 0, 0, 0, 0, 0, 0]
  map1 : xbsIndex_r3/ROM  depth=16  initVector=[0 4 2 6 1 5 3 7 8 12 10 14 9 13 11 15]  arith_type=Unsigned  n_bits=4  bin_pt=0  latency=0  init_zero=on  explicit_period=off  period=1  rst=off  init_reg=0  en=off  dbl_ovrd=off  show_param=off  distributed_mem=on  use_rpm=off  gen_core=off
      settings: xl_area=[0, 0, 0, 0, 0, 0, 0]
  post_sync_delay : xbsIndex_r3/Delay  latency=3  reg_retiming=off  explicit_period=off  period=1  en=off  accept_only_valid=off  init_zero=on  dbl_ovrd=off  show_param=off
      settings: xl_area=[0, 0, 0, 0, 0, 0, 0]
  pre_sync_delay : xbsIndex_r3/Delay  latency=0  reg_retiming=off  explicit_period=off  period=1  en=off  accept_only_valid=off  init_zero=on  dbl_ovrd=off  show_param=off
      settings: xl_area=[0, 0, 0, 0, 0, 0, 0]
  sync_delay_en : casper_library/Delays/sync_delay_en  DelayLen=16
      link override Constant: equ=P=C
      link override Constant1: equ=P=C
      link override Constant2: equ=P=C
      link override Constant3: equ=P=C
  sync_out : Outport
  valid : Outport  Port=2
  dout0 : Outport  Port=3
  wires:
  sync/1 -> Counter/1, pre_sync_delay/1
  en/1 -> Counter/2, sync_delay_en/2, delay_we/1
  Counter/1 -> Slice1/1, Slice2/1
  Slice1/1 -> delay_sel/1
  delay_sel/1 -> Mux/1
  Slice2/1 -> delay_d0/1, map1/1
  delay_d0/1 -> Mux/2
  pre_sync_delay/1 -> sync_delay_en/1
  sync_delay_en/1 -> post_sync_delay/1
  post_sync_delay/1 -> sync_out/1
  delay_we/1 -> delay_valid/1, bram0/3
  delay_valid/1 -> valid/1
  Mux/1 -> bram0/1
  din0/1 -> delay_din0/1
  delay_din0/1 -> bram0/2
  bram0/1 -> dout0/1
  map1/1 -> delay_map1/1
  delay_map1/1 -> Mux/3

== system casperdemo/Complex FFT and PFB/fft/fft_biplex0/biplex_cplx_unscrambler/reorder1 ==
  sync : Inport  Port=1  LatchInput=off
  en : Inport  Port=2  LatchInput=off
  din0 : Inport  Port=3  LatchInput=off
  Counter : xbsIndex_r3/Counter  cnt_type=Count Limited  n_bits=5  bin_pt=0  arith_type=Unsigned  start_count=0  cnt_to=31  cnt_by_val=1  operation=Up  explicit_period=off  period=1  load_pin=off  rst=on  en=on  dbl_ovrd=off  show_param=off  use_rpm=on  gen_core=off
      settings: xl_area=[0, 0, 0, 0, 0, 0, 0]
  Mux : xbsIndex_r3/Mux  inputs=2  precision=Full  arith_type="Signed  (2's comp)"  n_bits=8  bin_pt=2  quantization=Truncate  overflow=Wrap  latency=1  explicit_period=off  period=1  en=off  dbl_ovrd=off  show_param=off  mux_type=off  use_rpm=off  gen_core=off
      settings: xl_area=[0, 0, 0, 0, 0, 0, 0]
  Slice1 : xbsIndex_r3/Slice  mode=Upper Bit Location + Width  nbits=1  bit1=0  base1=MSB of Input  bit0=0  base0=LSB of Input  boolean_output=off  explicit_period=off  period=1  dbl_ovrd=off
  Slice2 : xbsIndex_r3/Slice  mode=Lower Bit Location + Width  nbits=4  bit1=0  base1=MSB of Input  bit0=0  base0=LSB of Input  boolean_output=off  explicit_period=off  period=1  dbl_ovrd=off
  bram0 : xbsIndex_r3/Single Port RAM  depth=16  initVector=sin(pi*(0:15)/16)  write_mode=Read Before Write  latency=2  init_zero=on  explicit_period=off  period=1  rst=off  init_reg=0  en=off  dbl_ovrd=off  show_param=off  distributed_mem=off  use_rpm=off  gen_core=off
      settings: xl_area=[0, 0, 0, 0, 0, 0, 0]
  delay_d0 : xbsIndex_r3/Delay  latency=0  reg_retiming=off  explicit_period=off  period=1  en=off  accept_only_valid=off  init_zero=on  dbl_ovrd=off  show_param=off
      settings: xl_area=[0, 0, 0, 0, 0, 0, 0]
  delay_din0 : xbsIndex_r3/Delay  latency=1  reg_retiming=off  explicit_period=off  period=1  en=off  accept_only_valid=off  init_zero=on  dbl_ovrd=off  show_param=off
      settings: xl_area=[0, 0, 0, 0, 0, 0, 0]
  delay_map1 : xbsIndex_r3/Delay  latency=0*map_latency  reg_retiming=off  explicit_period=off  period=1  en=off  accept_only_valid=off  init_zero=on  dbl_ovrd=off  show_param=off
      settings: xl_area=[0, 0, 0, 0, 0, 0, 0]
  delay_sel : xbsIndex_r3/Delay  latency=0  reg_retiming=off  explicit_period=off  period=1  en=off  accept_only_valid=off  init_zero=on  dbl_ovrd=off  show_param=off
      settings: xl_area=[0, 0, 0, 0, 0, 0, 0]
  delay_valid : xbsIndex_r3/Delay  latency=3  reg_retiming=off  explicit_period=off  period=1  en=off  accept_only_valid=off  init_zero=on  dbl_ovrd=off  show_param=off
      settings: xl_area=[0, 0, 0, 0, 0, 0, 0]
  delay_we : xbsIndex_r3/Delay  latency=0  reg_retiming=off  explicit_period=off  period=1  en=off  accept_only_valid=off  init_zero=on  dbl_ovrd=off  show_param=off
      settings: xl_area=[0, 0, 0, 0, 0, 0, 0]
  map1 : xbsIndex_r3/ROM  depth=16  initVector=[8 12 10 14 9 13 11 15 0 4 2 6 1 5 3 7]  arith_type=Unsigned  n_bits=4  bin_pt=0  latency=0  init_zero=on  explicit_period=off  period=1  rst=off  init_reg=0  en=off  dbl_ovrd=off  show_param=off  distributed_mem=on  use_rpm=off  gen_core=off
      settings: xl_area=[0, 0, 0, 0, 0, 0, 0]
  post_sync_delay : xbsIndex_r3/Delay  latency=3  reg_retiming=off  explicit_period=off  period=1  en=off  accept_only_valid=off  init_zero=on  dbl_ovrd=off  show_param=off
      settings: xl_area=[0, 0, 0, 0, 0, 0, 0]
  pre_sync_delay : xbsIndex_r3/Delay  latency=0  reg_retiming=off  explicit_period=off  period=1  en=off  accept_only_valid=off  init_zero=on  dbl_ovrd=off  show_param=off
      settings: xl_area=[0, 0, 0, 0, 0, 0, 0]
  sync_delay_en : casper_library/Delays/sync_delay_en  DelayLen=16
      link override Constant: equ=P=C
      link override Constant1: equ=P=C
      link override Constant2: equ=P=C
      link override Constant3: equ=P=C
  sync_out : Outport
  valid : Outport  Port=2
  dout0 : Outport  Port=3
  wires:
  sync/1 -> Counter/1, pre_sync_delay/1
  en/1 -> Counter/2, sync_delay_en/2, delay_we/1
  Counter/1 -> Slice1/1, Slice2/1
  Slice1/1 -> delay_sel/1
  delay_sel/1 -> Mux/1
  Slice2/1 -> delay_d0/1, map1/1
  delay_d0/1 -> Mux/2
  pre_sync_delay/1 -> sync_delay_en/1
  sync_delay_en/1 -> post_sync_delay/1
  post_sync_delay/1 -> sync_out/1
  delay_we/1 -> delay_valid/1, bram0/3
  delay_valid/1 -> valid/1
  Mux/1 -> bram0/1
  din0/1 -> delay_din0/1
  delay_din0/1 -> bram0/2
  bram0/1 -> dout0/1
  map1/1 -> delay_map1/1
  delay_map1/1 -> Mux/3

== system casperdemo/Complex FFT and PFB/pfb_fir/pol1_in1_last_tap/pfb_add_tree/adder_tree1 ==
  sync : Inport  Port=1  LatchInput=off
  din1 : Inport  Port=2  LatchInput=off
  din2 : Inport  Port=3  LatchInput=off
  din3 : Inport  Port=4  LatchInput=off
  din4 : Inport  Port=5  LatchInput=off
  addr1 : xbsIndex_r3/AddSub  mode=Addition  precision=Full  arith_type=Unsigned  n_bits=8  bin_pt=2  quantization=Truncate  overflow=Wrap  latency=1  explicit_period=off  period=1  use_carryin=off  use_carryout=off  en=off  dbl_ovrd=off  show_param=off  use_core=on  pipeline=on  use_rpm=on  gen_core=off
      settings: xl_area=[0, 0, 0, 0, 0, 0, 0]
  addr2 : xbsIndex_r3/AddSub  mode=Addition  precision=Full  arith_type=Unsigned  n_bits=8  bin_pt=2  quantization=Truncate  overflow=Wrap  latency=1  explicit_period=off  period=1  use_carryin=off  use_carryout=off  en=off  dbl_ovrd=off  show_param=off  use_core=on  pipeline=on  use_rpm=on  gen_core=off
      settings: xl_area=[0, 0, 0, 0, 0, 0, 0]
  addr3 : xbsIndex_r3/AddSub  mode=Addition  precision=Full  arith_type=Unsigned  n_bits=8  bin_pt=2  quantization=Truncate  overflow=Wrap  latency=1  explicit_period=off  period=1  use_carryin=off  use_carryout=off  en=off  dbl_ovrd=off  show_param=off  use_core=on  pipeline=on  use_rpm=on  gen_core=off
      settings: xl_area=[0, 0, 0, 0, 0, 0, 0]
  sync_delay : xbsIndex_r3/Delay  latency=2  reg_retiming=off  explicit_period=off  period=1  en=off  accept_only_valid=off  init_zero=on  dbl_ovrd=off  show_param=off
      settings: xl_area=[0, 0, 0, 0, 0, 0, 0]
  sync_out : Outport
  dout : Outport  Port=2
  wires:
  sync/1 -> sync_delay/1
  sync_delay/1 -> sync_out/1
  din1/1 -> addr1/1
  din2/1 -> addr1/2
  din3/1 -> addr2/1
  din4/1 -> addr2/2
  addr1/1 -> addr3/1
  addr2/1 -> addr3/2
  addr3/1 -> dout/1

== system casperdemo/Complex FFT and PFB/pfb_fir/pol1_in1_last_tap/pfb_add_tree/adder_tree2 ==
  sync : Inport  Port=1  LatchInput=off
  din1 : Inport  Port=2  LatchInput=off
  din2 : Inport  Port=3  LatchInput=off
  din3 : Inport  Port=4  LatchInput=off
  din4 : Inport  Port=5  LatchInput=off
  addr1 : xbsIndex_r3/AddSub  mode=Addition  precision=Full  arith_type=Unsigned  n_bits=8  bin_pt=2  quantization=Truncate  overflow=Wrap  latency=1  explicit_period=off  period=1  use_carryin=off  use_carryout=off  en=off  dbl_ovrd=off  show_param=off  use_core=on  pipeline=on  use_rpm=on  gen_core=off
      settings: xl_area=[0, 0, 0, 0, 0, 0, 0]
  addr2 : xbsIndex_r3/AddSub  mode=Addition  precision=Full  arith_type=Unsigned  n_bits=8  bin_pt=2  quantization=Truncate  overflow=Wrap  latency=1  explicit_period=off  period=1  use_carryin=off  use_carryout=off  en=off  dbl_ovrd=off  show_param=off  use_core=on  pipeline=on  use_rpm=on  gen_core=off
      settings: xl_area=[0, 0, 0, 0, 0, 0, 0]
  addr3 : xbsIndex_r3/AddSub  mode=Addition  precision=Full  arith_type=Unsigned  n_bits=8  bin_pt=2  quantization=Truncate  overflow=Wrap  latency=1  explicit_period=off  period=1  use_carryin=off  use_carryout=off  en=off  dbl_ovrd=off  show_param=off  use_core=on  pipeline=on  use_rpm=on  gen_core=off
      settings: xl_area=[0, 0, 0, 0, 0, 0, 0]
  sync_delay : xbsIndex_r3/Delay  latency=2  reg_retiming=off  explicit_period=off  period=1  en=off  accept_only_valid=off  init_zero=on  dbl_ovrd=off  show_param=off
      settings: xl_area=[0, 0, 0, 0, 0, 0, 0]
  sync_out : Outport
  dout : Outport  Port=2
  wires:
  sync/1 -> sync_delay/1
  sync_delay/1 -> sync_out/1
  din1/1 -> addr1/1
  din2/1 -> addr1/2
  din3/1 -> addr2/1
  din4/1 -> addr2/2
  addr1/1 -> addr3/1
  addr2/1 -> addr3/2
  addr3/1 -> dout/1

== system casperdemo/Complex FFT and PFB/pfb_fir/pol2_in1_last_tap/pfb_add_tree/adder_tree1 ==
  sync : Inport  Port=1  LatchInput=off
  din1 : Inport  Port=2  LatchInput=off
  din2 : Inport  Port=3  LatchInput=off
  din3 : Inport  Port=4  LatchInput=off
  din4 : Inport  Port=5  LatchInput=off
  addr1 : xbsIndex_r3/AddSub  mode=Addition  precision=Full  arith_type=Unsigned  n_bits=8  bin_pt=2  quantization=Truncate  overflow=Wrap  latency=1  explicit_period=off  period=1  use_carryin=off  use_carryout=off  en=off  dbl_ovrd=off  show_param=off  use_core=on  pipeline=on  use_rpm=on  gen_core=off
      settings: xl_area=[0, 0, 0, 0, 0, 0, 0]
  addr2 : xbsIndex_r3/AddSub  mode=Addition  precision=Full  arith_type=Unsigned  n_bits=8  bin_pt=2  quantization=Truncate  overflow=Wrap  latency=1  explicit_period=off  period=1  use_carryin=off  use_carryout=off  en=off  dbl_ovrd=off  show_param=off  use_core=on  pipeline=on  use_rpm=on  gen_core=off
      settings: xl_area=[0, 0, 0, 0, 0, 0, 0]
  addr3 : xbsIndex_r3/AddSub  mode=Addition  precision=Full  arith_type=Unsigned  n_bits=8  bin_pt=2  quantization=Truncate  overflow=Wrap  latency=1  explicit_period=off  period=1  use_carryin=off  use_carryout=off  en=off  dbl_ovrd=off  show_param=off  use_core=on  pipeline=on  use_rpm=on  gen_core=off
      settings: xl_area=[0, 0, 0, 0, 0, 0, 0]
  sync_delay : xbsIndex_r3/Delay  latency=2  reg_retiming=off  explicit_period=off  period=1  en=off  accept_only_valid=off  init_zero=on  dbl_ovrd=off  show_param=off
      settings: xl_area=[0, 0, 0, 0, 0, 0, 0]
  sync_out : Outport
  dout : Outport  Port=2
  wires:
  sync/1 -> sync_delay/1
  sync_delay/1 -> sync_out/1
  din1/1 -> addr1/1
  din2/1 -> addr1/2
  din3/1 -> addr2/1
  din4/1 -> addr2/2
  addr1/1 -> addr3/1
  addr2/1 -> addr3/2
  addr3/1 -> dout/1
